simulink model "demo"  (R2019a)
settings: Solver=ode2  StartTime=0.0  StopTime=inf  FixedStep=0.001  RelTol=1e-3  EnableMultiTasking=on
undefined symbols (not defined in the file): qc_get_step_size
libraries: quarc_library x5, xpcutilitieslib x1
settings Model: SimulationMode=external  Creator=user  LastModifiedBy=user
settings SolverCC: PositivePriorityOrder=on  AutoInsertRateTranBlk=on
settings RTWCC: SystemTargetFile=quarc_win64.tlc  TemplateMakefile=quarc_default_tmf  Description=QUARC Win64 Target
settings STFCustomTargetCC: TargetLangStandard=C99 (ISO)  ConcurrentExecutionCompliant=on  SystemTargetFile=quarc_win64.tlc
settings GRTTargetCC: TargetPreCompLibLocation=C:\PROGRA~3\QUARC\lib\2019a\win64\release  ParMdlRefBuildCompliant=off  CompOptLevelCompliant=off  CombineOutputUpdateFcns=off  MatFileLogging=off  CPPClassGenCompliant=off  GRTInterface=on  UseToolchainInfoCompliant=off  ExtMode=on  ExtModeMexFile=quarc_comm  ExtModeMexArgs='-w -d %d -uri %u -URI_Host tcpip://192.168.2.11:17201'

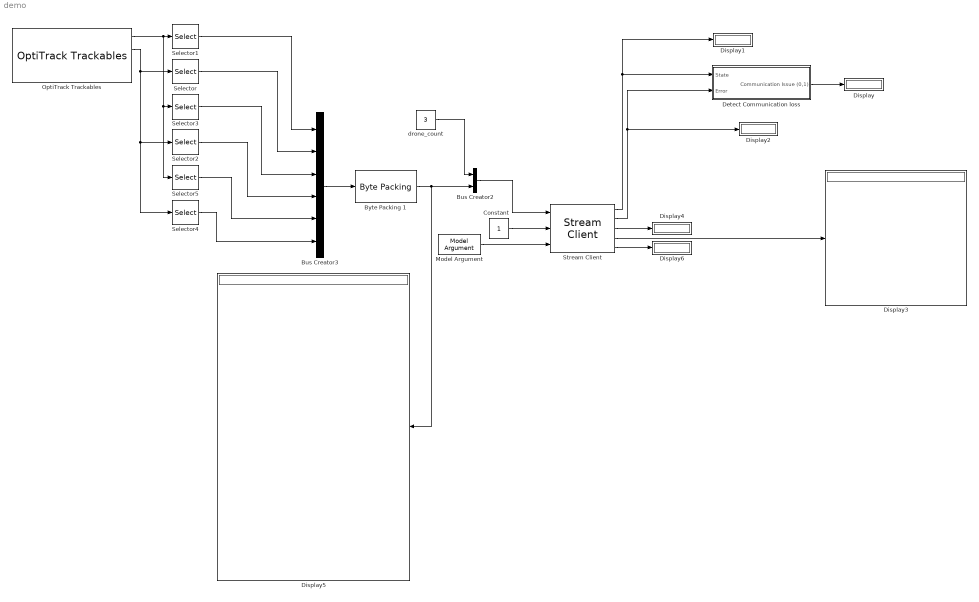
== system demo ==
  Bus Creator2 : BusCreator  Inputs=2
  Bus Creator3 : BusCreator  Inputs=6
  Byte Packing 1 : xpcutilitieslib/Byte Packing   MaskPackedDataType=uint8  MaskUnpackedDataTypes={'double'}  MaskAlignment=1
  Constant : Constant
  Detect Communication loss : Subsystem
  Display{,1..6} (7 alike) : Display
      Display5 settings: Format=hex (Stored Integer)  Decimation=7
  Model Argument : quarc_library/Sources/Signals/Model Argument  argument_name=URI_Host  has_value=on  data_type_mode=Specify via dialog  data_type=char  max_length=80  variable_size=off
      settings: AttributesFormatString=(-%<argument_name>)  SourceProductName=QUARC Targets
  OptiTrack Trackables : quarc_library/Devices/Third-Party/NaturalPoint/OptiTrack/OptiTrack Trackables  calibration_file=C:\Users\user\Desktop\Calibration Excellent (MeanErr 1.333 mm) 2021-01-06 6.cal  rigid_body_file=C:\Users\user\Desktop\RigidBody 04.tra  rigid_body_ids=[1,2,3]  sample_time=qc_get_step_size*10
      settings: SourceProductName=QUARC Targets
  Selector : Selector  InputPortWidth=12  IndexOptions=Index vector (dialog)  Indices=[1:4]  OutputSizes=1
  Selector1 : Selector  InputPortWidth=9  IndexOptions=Index vector (dialog)  Indices=[1:3]  OutputSizes=1
  Selector2 : Selector  InputPortWidth=12  IndexOptions=Index vector (dialog)  Indices=[5:8]  OutputSizes=1
  Selector3 : Selector  InputPortWidth=9  IndexOptions=Index vector (dialog)  Indices=[4:6]  OutputSizes=1
  Selector4 : Selector  InputPortWidth=12  IndexOptions=Index vector (dialog)  Indices=[9:12]  OutputSizes=1
  Selector5 : Selector  InputPortWidth=9  IndexOptions=Index vector (dialog)  Indices=[7:9]  OutputSizes=1
  Stream Client : quarc_library/Communications/Basic/Stream Client  uri_source=External input port  uri=tcpip://remotehost:18000  apply_uri_to_all_configs=on  send_buffer_size=1460  receive_buffer_size=1460  byte_order=big endian (Motorola - MSB first)  optimization=Minimum latency  send_options=Send most recent data  receive_options=Receive all data  default_value=zeros(1,36)  sample_time=0.01  active=off  implementation=Use blocking I/O in a separate thread  send_fifo_size=1000  receive_fifo_size=5000  send_priority=0  receive_priority=0  send_dimensions=off  receive_dimensions=off  max_dimensions=-1  data_type=double  type_expr=[double]
  drone_count : Constant  Value=3  OutDataTypeStr=uint8
  wires:
  Stream Client/5 -> Display6/1
  Byte Packing 1/1 -> Display5/1, Bus Creator2/2
  Bus Creator3/1 -> Byte Packing 1/1
  Stream Client/2 -> Detect Communication loss/2(Error), Display2/1
  Model Argument/1 -> Stream Client/3
  Bus Creator2/1 -> Stream Client/1
  drone_count/1 -> Bus Creator2/1
  Stream Client/4 -> Display3/1
  Detect Communication loss/1(Communication Issue (0,1)) -> Display/1
  Stream Client/3 -> Display4/1
  Constant/1 -> Stream Client/2
  Stream Client/1 -> Display1/1, Detect Communication loss/1(State)
  OptiTrack Trackables/2 -> Selector2/1, Selector4/1, Selector/1
  OptiTrack Trackables/1 -> Selector3/1, Selector5/1, Selector1/1
  Selector1/1 -> Bus Creator3/1
  Selector/1 -> Bus Creator3/2
  Selector3/1 -> Bus Creator3/3
  Selector2/1 -> Bus Creator3/4
  Selector5/1 -> Bus Creator3/5
  Selector4/1 -> Bus Creator3/6

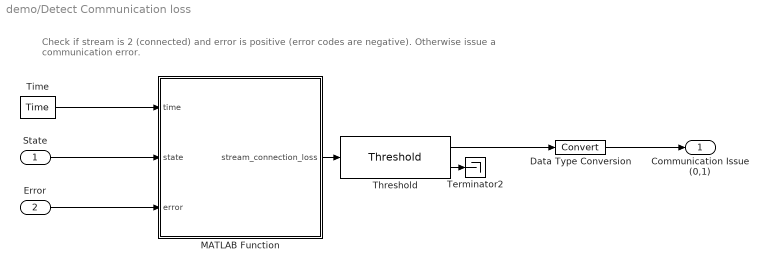
== system demo/Detect Communication loss ==
  note: Check if stream is 2 (connected) and error is positive (error codes are negative). Otherwise issue a communication error.
  State : Inport
  Error : Inport  Port=2
  Data Type Conversion : DataTypeConversion
  MATLAB Function : MATLAB Function  TreatAsAtomicUnit=on
  Terminator2 : Terminator
  Threshold : quarc_library/Discontinuities/Threshold  operator=>=  param_src=Specify via dialog  threshold=0.5  duration=0.1
      settings: SourceProductName=QUARC Targets
  Time : quarc_library/Sources/Time/Time  time_source=Wall clock  sample_time=qc_get_step_size
  Communication Issue (0,1) : Outport
  wires:
  Error/1 -> MATLAB Function/3(error)
  MATLAB Function/1(stream_connection_loss) -> Threshold/1
  State/1 -> MATLAB Function/2(state)
  Time/1 -> MATLAB Function/1(time)
  Threshold/2 -> Terminator2/1
  Data Type Conversion/1 -> Communication Issue (0,1)/1
  Threshold/1 -> Data Type Conversion/1

== matlab function demo/Detect Communication loss/MATLAB Function ==
  data: time input; stream_connection_loss output; state input; error input
function stream_connection_loss  = fcn(time, state, error)

stream_connection_loss = 0;
if time > 1
    if ~((state == 2)&&(error >= 0))
        % stream connection is not established correctly
        stream_connection_loss = 1;
    end
end
